simulink model "X8"  (R2020b)
settings: Solver=FixedStepAuto  StartTime=0.0  StopTime=Inf  FixedStep=1e-3  MinStep=0.0001  RelTol=1e-3  EnableMultiTasking=on
model workspace (MAT data in the model file):
  FaultMode : Simulink.Parameter (value not decoded)
values from neighbouring files (symbols this model uses):
  A = [ ... (first row only)    [calc_sys_long.m]
  C_L_delta_eInterpolation = Create_interpolation(C_L_delta_e_data,'C_L_delta_e_data')    [coeff_ctrl.m]
  F = K * (-(C_D_0 + C_D_alpha * alpha) * cos(alpha)      + (C_L_O + C_L_alpha * alpha)*sin(alpha)) - f_x    [calc_alpha.m]
  h0 = 1000    [init.m]
  input_source = 4    [runX8.m]
  input_source0 = 1    [runX8.m]
  input_step_time = 0    [runX8.m]
  J = @(v_a, omega) 2 * pi * v_a / (omega*obj.prop_diam)    [kalmanFilters.m]    (also in motor.m = 2*pi*Va/omega/prop_diam; motor_fault.m = c2 / omega)
  lat0 = 37.6205    [init.m]
  lon0 = -122.3815    [init.m]
  P = filter.P(i,i,k_0:k_1)    [filterTest.m]    (also in kalmanFilters.m = filter.P)
  p = rate(1) + wind(4)    [forces.m]    (also in forces_trim.m)
  q = rate(2) + wind(5)    [forces.m]    (also in forces_trim.m)
  r = rate(3) + wind(6)    [forces.m]    (also in forces_trim.m)
  T_elevon2ailelev = [1 1 ... (first row only)    [init.m]
  Ts = 0.01    [init.m]
  U_trim = [op.Inputs(1).u;op.Inputs(2).u;op.Inputs(3).u;op.Inputs(4).u]    [X8Trim.m]
  x0 = X_trim    [X8Trim.m]    (also in init.m = [eta_0', ny_0' zeros(1,6)]'; runX8.m = [      0                 0                    -h_ini        ; trimX8.m = [      37.5                 0                    -h_ini     )
symbols that are objects in the model workspace (value not decoded): FaultMode
undefined symbols (not defined in the file or in its folder): Friction, ia, ib, interp_C_D_alpha, interp_C_D_delta_e, interp_C_D_q, interp_C_L_alpha, interp_C_l_beta, interp_C_l_delta_a, interp_C_L_delta_e, interp_C_l_delta_r, interp_C_l_p, interp_C_L_q, interp_C_l_r, interp_C_m_alpha, interp_C_m_delta_e, interp_C_m_q, interp_C_n_beta, interp_C_n_delta_a, interp_C_n_p, interp_C_n_r, interp_C_Y_beta, interp_C_Y_delta_a, interp_C_Y_delta_r, interp_C_Y_p, interp_C_Y_r, Ion, JSBSim, Light, Lithium, Lls, MIL, Prop_param, Rascal110, Receive, Rs, Send, Standard_Devices, thetam, UDP_Protocol, wm, x0_stationary
libraries: simulink_extras x15, simulink x8, aerolibwind2 x4, sldrtlib x3, aerolibfltsims x3, aerolibactuator x3, sharedtransform x3, electricdrivelib x2, dspnetwork x1, aerolibnav x1, sharedutil x1, powerlib_meascontrol x1
(part 2 of 2)

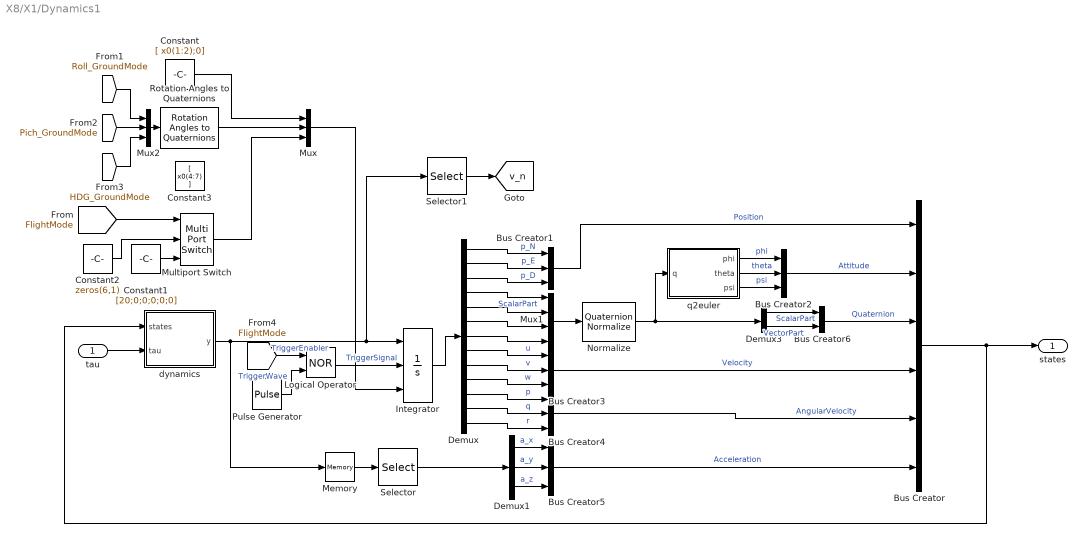
== system X8/X1/Dynamics1 ==
  tau : Inport
  Bus Creator : BusCreator  Inputs=6  OutDataTypeStr=Bus: States
  Bus Creator1 : BusCreator  Inputs=3  OutDataTypeStr=Bus: Position
  Bus Creator2 : BusCreator  Inputs=3  OutDataTypeStr=Bus: Attitude
  Bus Creator3 : BusCreator  Inputs=3  OutDataTypeStr=Bus: Velocity
  Bus Creator4 : BusCreator  Inputs=3  OutDataTypeStr=Bus: AngularVelocity
  Bus Creator5 : BusCreator  Inputs=3  OutDataTypeStr=Bus: Acceleration
  Bus Creator6 : BusCreator  Inputs=2  OutDataTypeStr=Bus: Quaternion
  Constant : Constant  Value=[ x0(1:2);0]
  Constant1 : Constant  Value=[20;0;0;0;0;0]
  Constant2 : Constant  Value=zeros(6,1)
  Constant3 : Constant  Value=[ x0(4:7) ]
  Demux : Demux  Outputs=13
  Demux1 : Demux  Outputs=3
  Demux3 : Demux  Outputs=[1,3]
  Integrator : Integrator  ExternalReset=either  InitialConditionSource=external  InitialCondition=x0_stationary(1:13)
  Logical Operator : Logic  Operator=NOR  AllPortsSameDT=off  OutDataTypeStr=boolean
  Memory : Memory
  Multiport Switch : MultiPortSwitch  DataPortOrder=Zero-based contiguous  Inputs=2  zeroidx=on
  Mux : Mux  Inputs=3
  Mux1 : Mux
  Mux2 : Mux  Inputs=3
  Normalize : sharedutil/Quaternion Normalize  aMode=aMode
      settings: SourceProductBaseCode=AE,PW,MT,UV,VE,VP
  Pulse Generator : DiscretePulseGenerator  PulseType=Time based  Period=0.2  PulseWidth=50
  Rotation Angles to Quaternions : sharedtransform/Rotation Angles to Quaternions  rotationOrder=XYZ  aMode=aMode
      settings: SourceProductBaseCode=AE,PW,MT,UV,VE,VP
  Selector : Selector  InputPortWidth=13  IndexOptions=Index vector (dialog)  Indices=8:10  OutputSizes=1
  Selector1 : Selector  InputPortWidth=13  IndexOptions=Index vector (dialog)  Indices=[1 2 3 11 12 13]  OutputSizes=1
  dynamics : MATLAB Function  TreatAsAtomicUnit=on
  q2euler : MATLAB Function  TreatAsAtomicUnit=on
  states : Outport  VectorParamsAs1DForOutWhenUnconnected=off
  tag scope: v_n=global
  wires:
  dynamics/1(y) -> Selector1/1, Integrator/1, Memory/1
  tau/1 -> dynamics/2(tau)
  Bus Creator/1 -> states/1, dynamics/1(states)
  Demux/2 -> Bus Creator1/2  "p_E"
  Demux/3 -> Bus Creator1/3  "p_D"
  Demux/1 -> Bus Creator1/1  "p_N"
  q2euler/2(theta) -> Bus Creator2/2  "theta"
  q2euler/3(psi) -> Bus Creator2/3  "psi"
  q2euler/1(phi) -> Bus Creator2/1  "phi"
  Demux/10 -> Bus Creator3/3  "w"
  Demux/8 -> Bus Creator3/1  "u"
  Demux/9 -> Bus Creator3/2  "v"
  Demux/11 -> Bus Creator4/1  "p"
  Demux/13 -> Bus Creator4/3  "r"
  Demux/12 -> Bus Creator4/2  "q"
  Bus Creator3/1 -> Bus Creator/4  "Velocity"
  Bus Creator1/1 -> Bus Creator/1  "Position"
  Bus Creator4/1 -> Bus Creator/5  "AngularVelocity"
  Bus Creator5/1 -> Bus Creator/6  "Acceleration"
  Selector/1 -> Demux1/1
  Demux1/1 -> Bus Creator5/1  "a_x"
  Demux1/2 -> Bus Creator5/2  "a_y"
  Demux1/3 -> Bus Creator5/3  "a_z"
  Demux/6 -> Mux1/3
  Demux/7 -> Mux1/4
  Demux/5 -> Mux1/2
  Normalize/1 -> q2euler/1(q), Demux3/1
  Integrator/1 -> Demux/1
  Demux3/1 -> Bus Creator6/1  "ScalarPart"
  Demux3/2 -> Bus Creator6/2  "VectorPart"
  Bus Creator6/1 -> Bus Creator/3  "Quaternion"
  Demux/4 -> Mux1/1  "ScalarPart"
  Bus Creator2/1 -> Bus Creator/2  "Attitude"
  Mux1/1 -> Normalize/1
  Memory/1 -> Selector/1
  [FlightMode] -> Multiport Switch/1
  Constant1/1 -> Multiport Switch/3
  Constant/1 -> Mux/1
  Mux2/1 -> Rotation Angles to Quaternions/1
  [Roll_GroundMode] -> Mux2/1
  [Pich_GroundMode] -> Mux2/2
  [HDG_GroundMode] -> Mux2/3
  Pulse Generator/1 -> Logical Operator/2  "TriggerWave"
  Logical Operator/1 -> Integrator/2  "TriggerSignal"
  [FlightMode] -> Logical Operator/1  "TriggerEnabler"
  Constant2/1 -> Multiport Switch/2
  Multiport Switch/1 -> Mux/3
  Mux/1 -> Integrator/3
  Rotation Angles to Quaternions/1 -> Mux/2
  Selector1/1 -> [v_n]

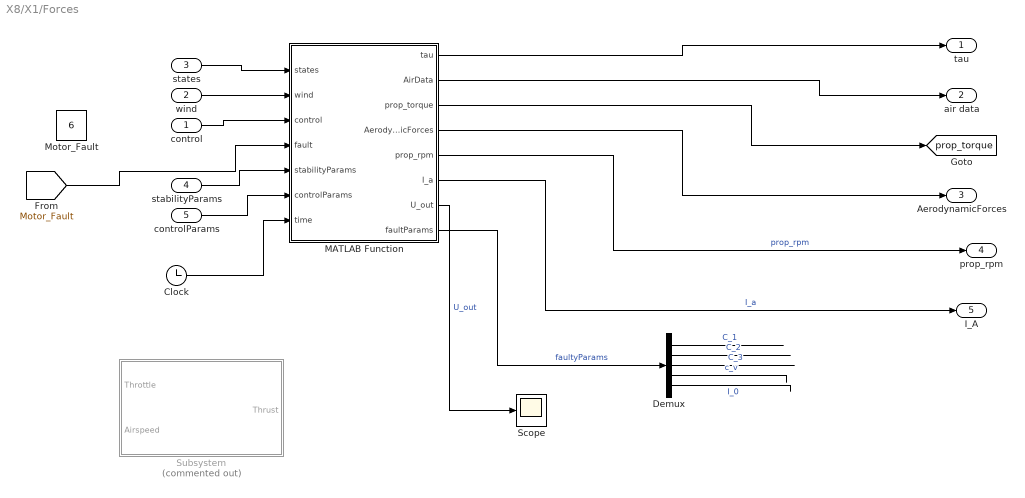
== system X8/X1/Forces ==
  control : Inport
  wind : Inport  Port=2
  states : Inport  Port=3
  stabilityParams : Inport  Port=4
  controlParams : Inport  Port=5
  Clock : Clock
  Demux : Demux  Outputs=5
  MATLAB Function : MATLAB Function  TreatAsAtomicUnit=on
  Motor_Fault : Constant  Value=6
  Scope : Scope
  Subsystem : Subsystem  Commented=on
  tau : Outport  VectorParamsAs1DForOutWhenUnconnected=off
  air data : Outport  Port=2  VectorParamsAs1DForOutWhenUnconnected=off
  AerodynamicForces : Outport  Port=3  VectorParamsAs1DForOutWhenUnconnected=off
  prop_rpm : Outport  Port=4  VectorParamsAs1DForOutWhenUnconnected=off
  I_A : Outport  Port=5  VectorParamsAs1DForOutWhenUnconnected=off
  tag scope: prop_torque=global
  wires:
  states/1 -> MATLAB Function/1(states)
  control/1 -> MATLAB Function/3(control)
  wind/1 -> MATLAB Function/2(wind)
  MATLAB Function/1(tau) -> tau/1
  MATLAB Function/3(prop_torque) -> [prop_torque]
  MATLAB Function/2(AirData) -> air data/1
  [Motor_Fault] -> MATLAB Function/4(fault)
  stabilityParams/1 -> MATLAB Function/5(stabilityParams)
  MATLAB Function/4(AerodynamicForces) -> AerodynamicForces/1
  controlParams/1 -> MATLAB Function/6(controlParams)
  MATLAB Function/5(prop_rpm) -> prop_rpm/1  "prop_rpm"
  MATLAB Function/6(I_a) -> I_A/1  "I_a"
  MATLAB Function/7(U_out) -> Scope/1  "U_out"
  Clock/1 -> MATLAB Function/7(time)
  MATLAB Function/8(faultParams) -> Demux/1  "faultyParams"
  Demux/1 -> ?  "C_1"
  Demux/2 -> ?  "C_2"
  Demux/3 -> ?  "C_3"
  Demux/4 -> ?  "c_v"
  Demux/5 -> ?  "I_0"

== system X8/X1/Terminate Function ==
  Event Listener : EventListener  DisableCoverage=on  EventType=Terminate  EventName=reset
  MATLAB Function : MATLAB Function  TreatAsAtomicUnit=on

== system X8/X1/wind model ==
  air data : Inport
  states : Inport  Port=2
  Bus Selector1 : BusSelector  OutputSignals=Va
  Bus Selector5 : BusSelector  OutputSignals=Position.p_D,Quaternion
  Dryden Wind Turbulence Model (Continuous (-q +r)) : aerolibwind2/Dryden Wind Turbulence Model  (Continuous (+q -r))  Commented=on  units=Metric (MKS)  spec=MIL-F-8785C  model=Discrete Dryden (+q -r)  W20=wind.speed  Wdeg=wind.dir  TurbProb=10^-2 - Light  L_high=533.4  Wingspan=P.b  ts=0.1  Seed=[23341 23342 23343 23344]  T_on=on
  Dryden Wind Turbulence Model (Discrete (-q +r)) : aerolibwind2/Dryden Wind Turbulence Model  (Continuous (+q -r))  units=Metric (MKS)  spec=MIL-F-8785C  model=Discrete Dryden (-q +r)  W20=3  Wdeg=wind.dir  TurbProb=10^-2 - Light  L_high=533.4  Wingspan=P.b  ts=1e-3  Seed=[23341 23342 23343 23344]  T_on=on
  Horizontal Wind Model : aerolibwind2/Horizontal Wind Model  units=Metric (MKS)  Vw_source=Internal  Vwind=3  W_source=Internal  Wdeg=wind.dir
      settings: SourceProductBaseCode=AE
  Mux : Mux  Inputs=2
  Quaternions to Direction Cosine Matrix : sharedtransform/Quaternions to  Direction Cosine Matrix  aMode=aMode
      settings: SourceProductBaseCode=AE,PW,MT,UV,VE,VP
  Sum : Sum  Inputs=|++
  Wind Shear Model : aerolibwind2/Wind Shear Model  Commented=on  units=Metric (MKS)  phase=Other  W_20=5  Wdeg=0
  down2h : Gain  Gain=-1
  gain shear wind : Gain  Commented=on  Gain=0
  gain shear wind3 : Gain
  zero wind1 : Constant  Commented=on  Value=zeros(3,1)
  wind : Outport  VectorParamsAs1DForOutWhenUnconnected=off
  wires:
  Bus Selector5/1 -> down2h/1  "<p_D>"
  Quaternions to Direction Cosine Matrix/1 -> Horizontal Wind Model/1, Dryden Wind Turbulence Model (Discrete (-q +r))/3, Wind Shear Model/2
  Bus Selector1/1 -> Dryden Wind Turbulence Model (Discrete (-q +r))/2  "<Va>"
  Bus Selector5/2 -> Quaternions to Direction Cosine Matrix/1  "<Quaternion>"
  air data/1 -> Bus Selector1/1
  states/1 -> Bus Selector5/1
  down2h/1 -> Wind Shear Model/1, Dryden Wind Turbulence Model (Discrete (-q +r))/1
  Wind Shear Model/1 -> gain shear wind/1
  Horizontal Wind Model/1 -> gain shear wind3/1
  Sum/1 -> Mux/1
  Dryden Wind Turbulence Model (Discrete (-q +r))/2 -> Mux/2
  ? -> ?
  Mux/1 -> wind/1
  gain shear wind3/1 -> Sum/1
  Dryden Wind Turbulence Model (Discrete (-q +r))/1 -> Sum/2

== system X8/X1/Actuators2/Actuator dynamics ==
  Demanded R elevon deflection : Inport
  "Demanded L elevon deflection " : Inport  Port=2
  Demanded rudder deflection1 : Inport  Port=3
  Demanded motor speed : Inport  Port=4
  Prop torque : Inport  Port=5
  Motor : Subsystem  Commented=through  mask{T=0.2, X0=x0(18)}
      mask prompts: T "Time constant"; X0 "Initial condition"
      mask DialogControl DescGroupVar Prompt: Motor model
      mask DialogControl DescTextVar Prompt: Simple first order motor model
  Saturation : Saturate  UpperLimit=P.aileronMax  LowerLimit=P.aileronMin
  Saturation1 : Saturate  UpperLimit=P.aileronMax  LowerLimit=P.aileronMin
  Servo and control surface dynamics L : aerolibactuator/Nonlinear Second-Order Actuator  Commented=through  wn_fin=P.servo.omega0  z_fin=P.servo.zeta  fin_max=P.servo.max_rad  fin_min=P.servo.min_rad  fin_maxrate=P.servo.rate_lim  fin_act_0=x0(16)  fin_act_vel=x0(17)
      settings: SourceProductBaseCode=AE
  Servo and control surface dynamics R : aerolibactuator/Nonlinear Second-Order Actuator  Commented=through  wn_fin=P.servo.omega0  z_fin=P.servo.zeta  fin_max=P.servo.max_rad  fin_min=P.servo.min_rad  fin_maxrate=P.servo.rate_lim  fin_act_0=x0(14)  fin_act_vel=x0(15)
      settings: SourceProductBaseCode=AE
  Servo and control surface dynamics1 : aerolibactuator/Nonlinear Second-Order Actuator  Commented=through  wn_fin=P.servo.omega0  z_fin=P.servo.zeta  fin_max=P.servo.max_rad  fin_min=P.servo.min_rad  fin_maxrate=P.servo.rate_lim  fin_act_0=P.servo.pos0  fin_act_vel=P.servo.rate0
      settings: SourceProductBaseCode=AE
  Subsystem : Subsystem  Commented=on
  Applied R elevon : Outport  VectorParamsAs1DForOutWhenUnconnected=off
  Applied L elevon : Outport  Port=2  VectorParamsAs1DForOutWhenUnconnected=off
  Applied rudder : Outport  Port=3  VectorParamsAs1DForOutWhenUnconnected=off
  Applied motor speed : Outport  Port=4  VectorParamsAs1DForOutWhenUnconnected=off
  wires:
  Servo and control surface dynamics R/1 -> Saturation/1
  Motor/1(n) -> Applied motor speed/1
  Servo and control surface dynamics1/1 -> Applied rudder/1
  Servo and control surface dynamics L/1 -> Saturation1/1
  Demanded rudder deflection1/1 -> Servo and control surface dynamics1/1
  Demanded motor speed/1 -> Motor/1(n_d)
  Demanded R elevon deflection/1 -> Servo and control surface dynamics R/1
  "Demanded L elevon deflection "/1 -> Servo and control surface dynamics L/1
  Saturation/1 -> Applied R elevon/1
  Saturation1/1 -> Applied L elevon/1

== system X8/X1/Actuators2/PWM lookup ==
  Rservo PWM : Inport
  Lservo : Inport  Port=2
  Rudder : Inport  Port=3
  thr pwm : Inport  Port=4
  1-D Lookup Table1 : Lookup_n-D  Commented=through  NumberOfTableDimensions=1  BreakpointsForDimension1=|  Table=|  InternalRulePriority=Speed  RndMeth=Simplest  InputSameDT=on
      BreakpointsForDimension1=|
      | [-20
      | -15
      | -10
      | 15
      | 20
      | 21.6]
      Table=|
      | [1260
      | 1400
      | 1480
      | 1770
      | 1880
      | 1920]
  1-D Lookup Table2 : Lookup_n-D  Commented=through  NumberOfTableDimensions=1  BreakpointsForDimension1=|  Table=|  InternalRulePriority=Speed  RndMeth=Simplest  InputSameDT=on
      BreakpointsForDimension1=|
      | [-20
      | -15
      | -10
      | 15
      | 20
      | 21.6]
      Table=|
      | [1260
      | 1400
      | 1480
      | 1770
      | 1880
      | 1920]
  1-D Lookup Table3 : Lookup_n-D  Commented=through  NumberOfTableDimensions=1  BreakpointsForDimension1=|  Table=|  InternalRulePriority=Speed  RndMeth=Simplest  InputSameDT=on
      BreakpointsForDimension1=|
      | [-20
      | -15
      | -10
      | 15
      | 20
      | 21.6]
      Table=|
      | [1260
      | 1400
      | 1480
      | 1770
      | 1880
      | 1920]
  Saturation{,1..3} (4 alike) : Saturate  Commented=through  UpperLimit=P.pwmMax  LowerLimit=P.pwmMin
  pwm to thrust : Lookup_n-D  Commented=through  NumberOfTableDimensions=1  BreakpointsForDimension1=[1000 2000]  Table=[0 1]  InternalRulePriority=Speed  RndMeth=Simplest  InputSameDT=on
  Rservo deflection : Outport  VectorParamsAs1DForOutWhenUnconnected=off
  Lservo deflection : Outport  Port=2  VectorParamsAs1DForOutWhenUnconnected=off
  rud deflection : Outport  Port=3  VectorParamsAs1DForOutWhenUnconnected=off
  thrust : Outport  Port=4  VectorParamsAs1DForOutWhenUnconnected=off
  wires:
  Saturation2/1 -> 1-D Lookup Table2/1
  1-D Lookup Table1/1 -> Rservo deflection/1
  pwm to thrust/1 -> thrust/1
  Rservo PWM/1 -> Saturation/1
  thr pwm/1 -> Saturation3/1
  Saturation1/1 -> 1-D Lookup Table3/1
  Saturation3/1 -> pwm to thrust/1
  Saturation/1 -> 1-D Lookup Table1/1
  Lservo/1 -> Saturation1/1
  Rudder/1 -> Saturation2/1
  1-D Lookup Table2/1 -> rud deflection/1
  1-D Lookup Table3/1 -> Lservo deflection/1

== system X8/X1/Actuators2/Scale to [-1..1] ==
  deflection : Inport
  Gain : Gain  Gain=1/P.aileronMax
  Saturation : Saturate  UpperLimit=1  LowerLimit=-1
  scaled deflection : Outport  VectorParamsAs1DForOutWhenUnconnected=off
  wires:
  deflection/1 -> Gain/1
  Gain/1 -> Saturation/1
  Saturation/1 -> scaled deflection/1

== system X8/X1/Actuators2/Scale to [0..1] ==
  prop speed : Inport
  Gain : Gain  Commented=through  Gain=1/P.motor.omega_max
  Saturation : Saturate  UpperLimit=1  LowerLimit=0
  scaled prop speed : Outport  VectorParamsAs1DForOutWhenUnconnected=off
  wires:
  prop speed/1 -> Gain/1
  Gain/1 -> Saturation/1
  Saturation/1 -> scaled prop speed/1

== system X8/X1/Calculate Stability Parameters/Subsystem ==
  alpha : Inport
  icing : Inport  Port=2
  2-D Lookup Table : Lookup_n-D  DataSpecification=Lookup table object  LookupTableObject=C_L_aInterpolation  BreakpointsForDimension1=C_L_delta_eInterpolation.Points(:,1)  BreakpointsForDimension2=C_L_delta_eInterpolation.Points(:,2)  BreakpointsForDimension1FirstPoint=4  BreakpointsForDimension2FirstPoint=2  IndexSearchMethod=Linear search  Table=C_L_delta_eInterpolation.Values  ExtrapMethod=Clip  InternalRulePriority=Speed  RndMeth=Simplest  InputSameDT=on
      settings: InputPortMap=u0,u1
  2-D Lookup Table1 : Lookup_n-D  DataSpecification=Lookup table object  LookupTableObject=C_L_qInterpolation  BreakpointsForDimension1=C_L_delta_eInterpolation.Points(:,1)  BreakpointsForDimension2=C_L_delta_eInterpolation.Points(:,2)  BreakpointsForDimension1FirstPoint=4  BreakpointsForDimension2FirstPoint=2  IndexSearchMethod=Linear search  Table=C_L_delta_eInterpolation.Values  InternalRulePriority=Speed  RndMeth=Simplest  InputSameDT=on
      settings: InputPortMap=u0,u1
  2-D Lookup Table2 : Lookup_n-D  DataSpecification=Lookup table object  LookupTableObject=C_D_aInterpolation  BreakpointsForDimension1=C_L_delta_eInterpolation.Points(:,1)  BreakpointsForDimension2=C_L_delta_eInterpolation.Points(:,2)  BreakpointsForDimension1FirstPoint=4  BreakpointsForDimension2FirstPoint=2  IndexSearchMethod=Linear search  Table=C_L_delta_eInterpolation.Values  InternalRulePriority=Speed  RndMeth=Simplest  InputSameDT=on
      settings: InputPortMap=u0,u1
  2-D Lookup Table3 : Lookup_n-D  DataSpecification=Lookup table object  LookupTableObject=C_D_qInterpolation  BreakpointsForDimension1=C_L_delta_eInterpolation.Points(:,1)  BreakpointsForDimension2=C_L_delta_eInterpolation.Points(:,2)  BreakpointsForDimension1FirstPoint=4  BreakpointsForDimension2FirstPoint=2  IndexSearchMethod=Linear search  Table=C_L_delta_eInterpolation.Values  InternalRulePriority=Speed  RndMeth=Simplest  InputSameDT=on
      settings: InputPortMap=u0,u1
  2-D Lookup Table4 : Lookup_n-D  DataSpecification=Lookup table object  LookupTableObject=C_m_qInterpolation  BreakpointsForDimension1=C_L_delta_eInterpolation.Points(:,1)  BreakpointsForDimension2=C_L_delta_eInterpolation.Points(:,2)  BreakpointsForDimension1FirstPoint=4  BreakpointsForDimension2FirstPoint=2  IndexSearchMethod=Linear search  Table=C_L_delta_eInterpolation.Values  InternalRulePriority=Speed  RndMeth=Simplest  InputSameDT=on
      settings: InputPortMap=u0,u1
  2-D Lookup Table5 : Lookup_n-D  DataSpecification=Lookup table object  LookupTableObject=C_m_aInterpolation  BreakpointsForDimension1=C_L_delta_eInterpolation.Points(:,1)  BreakpointsForDimension2=C_L_delta_eInterpolation.Points(:,2)  BreakpointsForDimension1FirstPoint=4  BreakpointsForDimension2FirstPoint=2  IndexSearchMethod=Linear search  Table=C_L_delta_eInterpolation.Values  InternalRulePriority=Speed  RndMeth=Simplest  InputSameDT=on
      settings: InputPortMap=u0,u1
  Bus Creator : BusCreator  Inputs=6
  Out1 : Outport  VectorParamsAs1DForOutWhenUnconnected=off
  wires:
  Bus Creator/1 -> Out1/1
  2-D Lookup Table/1 -> Bus Creator/1  "C_L_alpha"
  alpha/1 -> 2-D Lookup Table4/1, 2-D Lookup Table5/1, 2-D Lookup Table3/1, 2-D Lookup Table2/1, 2-D Lookup Table1/1, 2-D Lookup Table/1
  icing/1 -> 2-D Lookup Table3/2, 2-D Lookup Table5/2, 2-D Lookup Table4/2, 2-D Lookup Table2/2, 2-D Lookup Table1/2, 2-D Lookup Table/2
  2-D Lookup Table1/1 -> Bus Creator/2  "C_L_q"
  2-D Lookup Table2/1 -> Bus Creator/3  "C_D_alpha"
  2-D Lookup Table3/1 -> Bus Creator/4  "C_D_q"
  2-D Lookup Table5/1 -> Bus Creator/5  "C_m_alpha"
  2-D Lookup Table4/1 -> Bus Creator/6  "C_m_q"

== system X8/X1/Calculate Stability Parameters/Subsystem1 ==
  beta : Inport
  icing : Inport  Port=2
  2-D Lookup Table : Lookup_n-D  DataSpecification=Lookup table object  LookupTableObject=C_Y_bInterpolation  BreakpointsForDimension1=C_L_delta_eInterpolation.Points(:,1)  BreakpointsForDimension2=C_L_delta_eInterpolation.Points(:,2)  BreakpointsForDimension1FirstPoint=4  BreakpointsForDimension2FirstPoint=2  IndexSearchMethod=Linear search  Table=C_L_delta_eInterpolation.Values  InternalRulePriority=Speed  RndMeth=Simplest  InputSameDT=on
      settings: InputPortMap=u0,u1
  2-D Lookup Table1 : Lookup_n-D  DataSpecification=Lookup table object  LookupTableObject=C_Y_pInterpolation  BreakpointsForDimension1=C_L_delta_eInterpolation.Points(:,1)  BreakpointsForDimension2=C_L_delta_eInterpolation.Points(:,2)  BreakpointsForDimension1FirstPoint=4  BreakpointsForDimension2FirstPoint=2  IndexSearchMethod=Linear search  Table=C_L_delta_eInterpolation.Values  InternalRulePriority=Speed  RndMeth=Simplest  InputSameDT=on
      settings: InputPortMap=u0,u1
  2-D Lookup Table2 : Lookup_n-D  DataSpecification=Lookup table object  LookupTableObject=C_Y_rInterpolation  BreakpointsForDimension1=C_L_delta_eInterpolation.Points(:,1)  BreakpointsForDimension2=C_L_delta_eInterpolation.Points(:,2)  BreakpointsForDimension1FirstPoint=4  BreakpointsForDimension2FirstPoint=2  IndexSearchMethod=Linear search  Table=C_L_delta_eInterpolation.Values  InternalRulePriority=Speed  RndMeth=Simplest  InputSameDT=on
      settings: InputPortMap=u0,u1
  2-D Lookup Table3 : Lookup_n-D  DataSpecification=Lookup table object  LookupTableObject=C_l_bInterpolation  BreakpointsForDimension1=C_L_delta_eInterpolation.Points(:,1)  BreakpointsForDimension2=C_L_delta_eInterpolation.Points(:,2)  BreakpointsForDimension1FirstPoint=4  BreakpointsForDimension2FirstPoint=2  IndexSearchMethod=Linear search  Table=C_L_delta_eInterpolation.Values  InternalRulePriority=Speed  RndMeth=Simplest  InputSameDT=on
      settings: InputPortMap=u0,u1
  2-D Lookup Table4 : Lookup_n-D  DataSpecification=Lookup table object  LookupTableObject=C_l_rInterpolation  BreakpointsForDimension1=C_L_delta_eInterpolation.Points(:,1)  BreakpointsForDimension2=C_L_delta_eInterpolation.Points(:,2)  BreakpointsForDimension1FirstPoint=4  BreakpointsForDimension2FirstPoint=2  IndexSearchMethod=Linear search  Table=C_L_delta_eInterpolation.Values  InternalRulePriority=Speed  RndMeth=Simplest  InputSameDT=on
      settings: InputPortMap=u0,u1
  2-D Lookup Table5 : Lookup_n-D  DataSpecification=Lookup table object  LookupTableObject=C_l_pInterpolation  BreakpointsForDimension1=C_L_delta_eInterpolation.Points(:,1)  BreakpointsForDimension2=C_L_delta_eInterpolation.Points(:,2)  BreakpointsForDimension1FirstPoint=4  BreakpointsForDimension2FirstPoint=2  IndexSearchMethod=Linear search  Table=C_L_delta_eInterpolation.Values  InternalRulePriority=Speed  RndMeth=Simplest  InputSameDT=on
      settings: InputPortMap=u0,u1
  2-D Lookup Table6 : Lookup_n-D  DataSpecification=Lookup table object  LookupTableObject=C_n_bInterpolation  BreakpointsForDimension1=C_L_delta_eInterpolation.Points(:,1)  BreakpointsForDimension2=C_L_delta_eInterpolation.Points(:,2)  BreakpointsForDimension1FirstPoint=4  BreakpointsForDimension2FirstPoint=2  IndexSearchMethod=Linear search  Table=C_L_delta_eInterpolation.Values  InternalRulePriority=Speed  RndMeth=Simplest  InputSameDT=on
      settings: InputPortMap=u0,u1
  2-D Lookup Table7 : Lookup_n-D  DataSpecification=Lookup table object  LookupTableObject=C_n_pInterpolation  BreakpointsForDimension1=C_L_delta_eInterpolation.Points(:,1)  BreakpointsForDimension2=C_L_delta_eInterpolation.Points(:,2)  BreakpointsForDimension1FirstPoint=4  BreakpointsForDimension2FirstPoint=2  IndexSearchMethod=Linear search  Table=C_L_delta_eInterpolation.Values  InternalRulePriority=Speed  RndMeth=Simplest  InputSameDT=on
      settings: InputPortMap=u0,u1
  2-D Lookup Table8 : Lookup_n-D  DataSpecification=Lookup table object  LookupTableObject=C_n_rInterpolation  BreakpointsForDimension1=C_L_delta_eInterpolation.Points(:,1)  BreakpointsForDimension2=C_L_delta_eInterpolation.Points(:,2)  BreakpointsForDimension1FirstPoint=4  BreakpointsForDimension2FirstPoint=2  IndexSearchMethod=Linear search  Table=C_L_delta_eInterpolation.Values  InternalRulePriority=Speed  RndMeth=Simplest  InputSameDT=on
      settings: InputPortMap=u0,u1
  Bus Creator : BusCreator  Inputs=9
  Out1 : Outport  VectorParamsAs1DForOutWhenUnconnected=off
  wires:
  Bus Creator/1 -> Out1/1
  icing/1 -> 2-D Lookup Table/2, 2-D Lookup Table6/2, 2-D Lookup Table7/2, 2-D Lookup Table8/2, 2-D Lookup Table4/2, 2-D Lookup Table5/2, 2-D Lookup Table3/2, 2-D Lookup Table2/2, 2-D Lookup Table1/2
  2-D Lookup Table1/1 -> Bus Creator/2  "C_Y_p"
  beta/1 -> 2-D Lookup Table5/1, 2-D Lookup Table8/1, 2-D Lookup Table7/1, 2-D Lookup Table6/1, 2-D Lookup Table4/1, 2-D Lookup Table3/1, 2-D Lookup Table2/1, 2-D Lookup Table1/1, 2-D Lookup Table/1
  2-D Lookup Table2/1 -> Bus Creator/3  "C_Y_r"
  2-D Lookup Table/1 -> Bus Creator/1  "C_Y_beta"
  2-D Lookup Table5/1 -> Bus Creator/5  "C_l_p"
  2-D Lookup Table3/1 -> Bus Creator/4  "C_l_beta"
  2-D Lookup Table4/1 -> Bus Creator/6  "C_l_r"
  2-D Lookup Table6/1 -> Bus Creator/7  "C_n_beta"
  2-D Lookup Table7/1 -> Bus Creator/8  "C_n_p"
  2-D Lookup Table8/1 -> Bus Creator/9  "C_n_r"

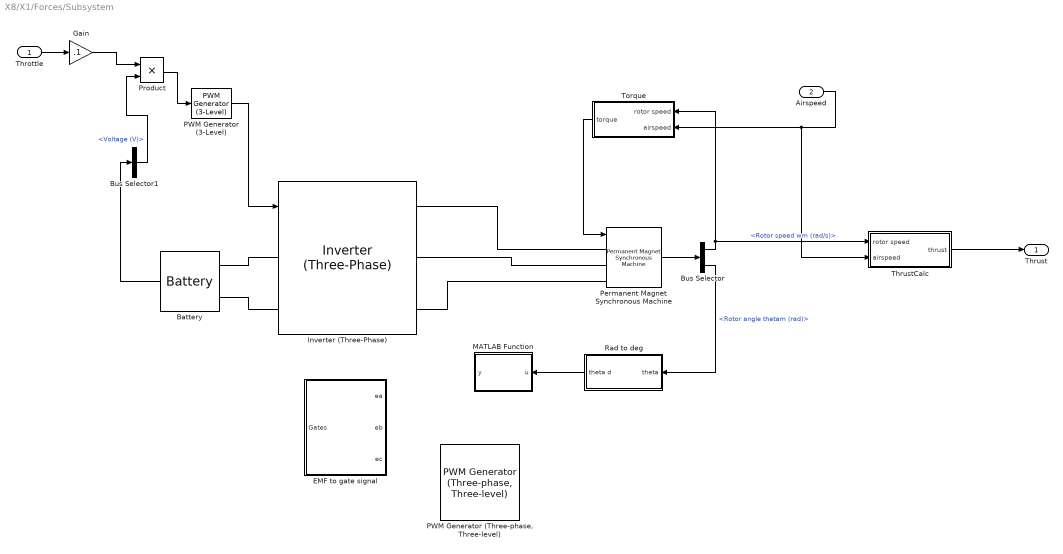
== system X8/X1/Forces/Subsystem ==
  Throttle : Inport
  Airspeed : Inport  Port=2
  Battery : electricdrivelib/Extra Sources/Battery  BatType=Lithium-Ion  ShowTempParam=off  ThermalPreset=no  ShowAgeParam=off  NomV=14  NomQ=1000  SOC=100  Batt_Tr=30  PresetModel=on  MaxQ=1000  MinV=10.5  FullV=16.2958  Dis_rate=434.7826  R=0.00014  Normal_OP=904.3478  expZone="[15.1254      49.1304]"  current=[6.5 13 32.5]  Units=Time  Tci=20  NomT=20  T2=-30  MaxQ2=4.8  FullV2=7.1  Normal_OP2=5.655  expZone2="[6.58           1]"  Rca=0.6  ti=2000  Dp=0  Neq0=0  Tsim=1e6  Ta1=25  Qeol=5.4*0.9  Reol=0.013333*1.2  Char_age=[2.3478, 3]  Dis_age=[2.3478, 10]  N1=1500  N2=10500  N3=1000  N4=1400  Ta2=45  N5=950
  Bus Selector : BusSelector  OutputSignals=Rotor speed wm (rad/s),Rotor angle thetam (rad)
  Bus Selector1 : BusSelector  OutputSignals=Voltage (V)
  EMF to gate signal : Subsystem
  Gain : Gain  Gain=.1
  Inverter (Three-Phase) : electricdrivelib/Fundamental Drive Blocks/Inverter (Three-Phase)  LabelModeActiveChoice=Detailed  detailLevel=Detailed  driveType=Brushless DC  Ts=2e-6  SnubberResistance=10e3  SnubberCapacitance=inf  Device=MOSFET / Diodes  Ron=1e-3  ForwardVoltages=[1.2,1.2]  GTOparameters=[1e-6,2e-6]  IGBTparameters=[1e-6,2e-6]  Measurements=All voltages and currents  converterType=Inverter  SourceFrequency=60  ReferenceFrame=Rotor  dqInductances=[8.5e-3,8.5e-3]  Inductance=8.5e-3  Ls=0  Resistance=0.2  Flux=0.175  Stator_sm=[2.01e-3,4.289e-4,4.477e-3,1.354e-3]  Stator_im=[14.85e-3,0.3027e-3]  Rotor=[9.295e-3,0.3027e-3]  Lm=10.46e-3  p=4
      settings: AttributesFormatString=%<BlockChoice>  SourceProductBaseCode=PS
  MATLAB Function : MATLAB Function  TreatAsAtomicUnit=on
  PWM Generator (3-Level) : powerlib_meascontrol/Pulse & Signal Generators/PWM Generator (3-Level)  ModulatorType=Three-phase bridge (12 pulses)  ModulatorMode=Unsynchronized  nF=27  Fc=27*60  ModulatingSignals=off  m=0.8  Freq=60  Phase=0  Ts=0
      settings: SourceProductBaseCode=PS
  "PWM Generator (Three-phase, Three-level)" : pePwmGeneratorThreeLevel/PWM Generator (Three-phase, Three-level)  CPWMMode=SPWM: sinusoidal PWM  fsw=1e3  Ts=5e-5
      settings: SourceProductBaseCode=PS  SamplingMode=Natural
  Permanent Magnet Synchronous Machine : powerlib/Machines/Permanent Magnet Synchronous Machine  NbPhases=3  FluxDistribution=Trapezoidal  RotorType=Round  MechanicalLoad=Torque Tm  PresetModel=No  ShowDetailedParameters=on  MeasurementBus=off  Resistance=Rs  Inductance=Lls  dqInductances=[8.5e-3,8.5e-3]  La=0.000835  MachineConstant=Flux linkage established by magnets (V.s)  Flux=0.175  VoltageCst=146.6077  TorqueCst=1.4  Flat=Flat  Mechanical=[J,Friction,p]  PolePairs=4  InitialConditions=[wm,thetam,ia,ib]  InitialConditions5ph=[0 0 0 0 0 0]  RefAngle=90 degrees behind phase A axis (modified Park)  IterativeDiscreteModel=Trapezoidal non iterative  TsBlock=-1  TsPowergui=0
  Product : Product
  Rad to deg : Subsystem
  ThrustCalc : Subsystem
  Torque : Subsystem
  Thrust : Outport  VectorParamsAs1DForOutWhenUnconnected=off
  wires:
  Permanent Magnet Synchronous Machine/1 -> Bus Selector/1
  Bus Selector/1 -> Torque/1(rotor speed), ThrustCalc/1(rotor speed)  "<Rotor speed wm (rad/s)>"
  PWM Generator (3-Level)/1 -> Inverter (Three-Phase)/1
  Battery/1 -> Bus Selector1/1
  Product/1 -> PWM Generator (3-Level)/1
  Bus Selector1/1 -> Product/2  "<Voltage (V)>"
  Throttle/1 -> Gain/1
  Gain/1 -> Product/1
  Torque/1(torque) -> Permanent Magnet Synchronous Machine/1
  ThrustCalc/1(thrust) -> Thrust/1
  Airspeed/1 -> ThrustCalc/2(airspeed), Torque/2(airspeed)
  Bus Selector/2 -> Rad to deg/1(theta)  "<Rotor angle thetam (rad)>"
  Rad to deg/1(theta d) -> MATLAB Function/1(u)
  connections:
  Battery/LConn1 -- Inverter (Three-Phase)/LConn1
  Battery/LConn2 -- Inverter (Three-Phase)/LConn2
  Inverter (Three-Phase)/RConn1 -- Permanent Magnet Synchronous Machine/LConn1
  Inverter (Three-Phase)/RConn2 -- Permanent Magnet Synchronous Machine/LConn2
  Inverter (Three-Phase)/RConn3 -- Permanent Magnet Synchronous Machine/LConn3

== system X8/X1/Actuators2/Actuator dynamics/Motor ==
  n_d : Inport
  1/T : Gain  Gain=1/T
  Integrator : Integrator  InitialCondition=X0  ContinuousStateAttributes='throttle'
  Sum : Sum  Inputs=|+-
  n : Outport  VectorParamsAs1DForOutWhenUnconnected=off
  wires:
  Integrator/1 -> n/1, Sum/2
  n_d/1 -> Sum/1
  Sum/1 -> 1/T/1
  1/T/1 -> Integrator/1

== system X8/X1/Actuators2/Actuator dynamics/Subsystem ==
  In1 : Inport
  In2 : Inport  Port=2
  1/J_prop : Gain  Gain=1/P.J_prop  SaturateOnIntegerOverflow=on  OutDataTypeStr=Inherit: Same as input  ParamDataTypeStr=Inherit: Same as input
  Demand limits : Saturate  UpperLimit=1  LowerLimit=0
  Integrator : Integrator  InitialCondition=0.5
  Kp : Gain  SaturateOnIntegerOverflow=on  OutDataTypeStr=Inherit: Same as input  ParamDataTypeStr=Inherit: Same as input
  Kp1 : Gain  Gain=-1  SaturateOnIntegerOverflow=on  OutDataTypeStr=Inherit: Same as input  ParamDataTypeStr=Inherit: Same as input
  Sum2 : Sum  Inputs=-+|  InputSameDT=on  SaturateOnIntegerOverflow=on  OutDataTypeStr=Inherit: Same as first input
  Sum3 : Sum  Inputs=|+-  InputSameDT=on  SaturateOnIntegerOverflow=on  OutDataTypeStr=Inherit: Same as first input
  Torque limit : Saturate  UpperLimit=P.motor.torque_max  LowerLimit=0  ZeroCross=off
  Transport Delay : TransportDelay  DelayTime=0.001  PadeOrder=1
  Applied motor speed : Outport  VectorParamsAs1DForOutWhenUnconnected=off
  wires:
  Demand limits/1 -> Sum3/1
  Sum3/1 -> Kp/1
  Integrator/1 -> Applied motor speed/1, Sum3/2
  Torque limit/1 -> Sum2/2
  Sum2/1 -> 1/J_prop/1
  1/J_prop/1 -> Integrator/1
  Kp/1 -> Torque limit/1
  In1/1 -> Kp1/1
  In2/1 -> Transport Delay/1
  Transport Delay/1 -> Demand limits/1
  Kp1/1 -> Sum2/1

== system X8/X1/Forces/Subsystem/EMF to gate signal ==
  ea : Inport
  eb : Inport  Port=2
  ec : Inport  Port=3
  Compare To Zero : simulink/Logic and Bit Operations/Compare To Zero  relop=>  OutDataTypeStr=boolean  ZeroCross=off
  Compare To Zero1 : simulink/Logic and Bit Operations/Compare To Zero  relop=<  OutDataTypeStr=boolean  ZeroCross=off
  Compare To Zero2 : simulink/Logic and Bit Operations/Compare To Zero  relop=>  OutDataTypeStr=boolean  ZeroCross=off
  Compare To Zero3 : simulink/Logic and Bit Operations/Compare To Zero  relop=<  OutDataTypeStr=boolean  ZeroCross=off
  Compare To Zero4 : simulink/Logic and Bit Operations/Compare To Zero  relop=>  OutDataTypeStr=boolean  ZeroCross=off
  Compare To Zero5 : simulink/Logic and Bit Operations/Compare To Zero  relop=<  OutDataTypeStr=boolean  ZeroCross=off
  Mux3 : Mux  Inputs=6
  Gates : Outport  VectorParamsAs1DForOutWhenUnconnected=off
  wires:
  Mux3/1 -> Gates/1
  ea/1 -> Compare To Zero/1, Compare To Zero1/1
  eb/1 -> Compare To Zero2/1, Compare To Zero3/1
  ec/1 -> Compare To Zero4/1, Compare To Zero5/1
  Compare To Zero/1 -> Mux3/1
  Compare To Zero1/1 -> Mux3/2
  Compare To Zero2/1 -> Mux3/3
  Compare To Zero3/1 -> Mux3/4
  Compare To Zero4/1 -> Mux3/5
  Compare To Zero5/1 -> Mux3/6

== system X8/X1/Forces/Subsystem/Rad to deg ==
  theta : Inport
  Trigonometric Function : Trigonometry
  Trigonometric Function1 : Trigonometry  Operator=cos
  Trigonometric Function2 : Trigonometry  Operator=atan2
  rad2deg : Gain  Gain=180/pi  SaturateOnIntegerOverflow=on  OutDataTypeStr=Inherit: Same as input  ParamDataTypeStr=Inherit: Same as input
  theta d : Outport  VectorParamsAs1DForOutWhenUnconnected=off
  wires:
  theta/1 -> Trigonometric Function/1, Trigonometric Function1/1
  Trigonometric Function/1 -> Trigonometric Function2/1
  Trigonometric Function1/1 -> Trigonometric Function2/2
  Trigonometric Function2/1 -> rad2deg/1
  rad2deg/1 -> theta d/1

== system X8/X1/Forces/Subsystem/ThrustCalc ==
  rotor speed : Inport
  airspeed : Inport  Port=2
  Divide : Product  Inputs=*/
  Divide1 : Product  Inputs=**
  Gain : Gain  Gain=2*pi
  Gain1 : Gain  Gain=Prop_param.C_T_0
  Gain2 : Gain  Gain=Prop_param.C_T_J
  Math Function : Math  Operator=square  SignedPower=on  SaturateOnIntegerOverflow=on
  Sum : Sum
  thrust : Outport  VectorParamsAs1DForOutWhenUnconnected=off
  wires:
  rotor speed/1 -> Math Function/1, Divide/2
  airspeed/1 -> Gain/1
  Gain/1 -> Divide/1
  Divide/1 -> Divide1/1  "J"
  Sum/1 -> thrust/1
  Math Function/1 -> Divide1/2, Gain1/1
  Divide1/1 -> Gain2/1  "J"
  Gain2/1 -> Sum/1
  Gain1/1 -> Sum/2

== system X8/X1/Forces/Subsystem/Torque ==
  rotor speed : Inport
  airspeed : Inport  Port=2
  Derivative : Derivative
  Divide : Product  Inputs=*/
  Divide1 : Product  Inputs=**
  Gain : Gain  Gain=2*pi
  Gain1 : Gain  Gain=Prop_param.C_W_0
  Gain2 : Gain  Gain=Prop_param.C_W_J
  Gain3 : Gain  Gain=Prop_param.c_v
  Gain4 : Gain  Gain=Prop_param.J
  Math Function : Math  Operator=square  SignedPower=on  SaturateOnIntegerOverflow=on
  Sum : Sum  Inputs=++++
  torque : Outport  VectorParamsAs1DForOutWhenUnconnected=off
  wires:
  rotor speed/1 -> Derivative/1, Math Function/1, Gain3/1, Divide/2
  airspeed/1 -> Gain/1
  Gain/1 -> Divide/1
  Divide/1 -> Divide1/1  "J"
  Sum/1 -> torque/1
  Math Function/1 -> Divide1/2, Gain1/1
  Gain1/1 -> Sum/3
  Divide1/1 -> Gain2/1  "J"
  Gain2/1 -> Sum/2
  Gain3/1 -> Sum/1
  Derivative/1 -> Gain4/1
  Gain4/1 -> Sum/4

== matlab function X8/MATLAB Function ==
  data: t input; icing output
function icing = fcn(t)
    % Some icing model. 
    % icing = 0..1 
    
    NOICE_PERIOD = 30;
    ICING_TIME = 30;
    MAX_ICING = 1; 
    
    if t < NOICE_PERIOD
        icing = 0; 
    elseif t < NOICE_PERIOD + ICING_TIME
        icing = MAX_ICING * (t - NOICE_PERIOD) / ICING_TIME; 
    else
        icing = MAX_ICING; 
    end
end

== matlab function X8/X1/Forces/Subsystem/MATLAB Function ==
  data: u input; y output
function y=emfg(u)
if (u>-180)&&(u<=-120)
    y=[-1;0;1];
elseif(u>-120)&&(u<=-60)
    y=[0;-1;1];
elseif(u>-60)&&(u<=0)
    y=[1;-1;0];
elseif(u>0)&&(u<=60)
    y=[1;0;-1];
elseif(u>60)&&(u<=120)
    y=[0;1;-1];
elseif(u>120)&&(u<=180)
    y=[-1;1;0];
end
y =[y(1)>0;y(1)<0;y(2)>0;y(2)<0;y(3)>0;y(3)<0];

== matlab function X8/X1/Send Dune Airflow1 ==
  settings: updateMethod=DISCRETE  sampleTime=0.1
  data: Va input; AoA input; SSA input; wind_n input
function rcv_airflow(Va,AoA,SSA,wind_n)
coder.extrinsic('-sync:on','send_airflow_dune');
send_airflow_dune(Va,AoA,SSA,wind_n,0);

== matlab function X8/Motor Fault ==
  settings: updateMethod=DISCRETE
  data: model input; y output; mode input
function y  = fcn(model, mode)
    y = mode * model;
end

== matlab function X8/X1/Terminate Function/MATLAB Function ==
function fcn()
coder.extrinsic('-sync:on','rcv_airflow_dune');
coder.extrinsic('-sync:on','send_airflow_dune');
send_airflow_dune(0,0,0,1);
[~,~,~]=rcv_airflow_dune(1);

end

== matlab function X8/Ardupilot SITL receive/MATLAB Function ==
  data: motors output
function motors = fcn()
motors = zeros(16 ,1);
coder.extrinsic('-sync:on','simReceive');
motors = simReceive();
end

== matlab function X8/Ardupilot SITL send/MATLAB Function ==
  data: Va input; u_r output; alpha input; beta input
function u_r = fcn(Va,alpha,beta)

u_r = Va*cos(alpha)*cos(beta);

== matlab function X8/Ardupilot SITL send/MATLAB Function1 ==
  data: u input; y output
function y  = fcn(u)

y = Rquat(u);

== matlab function X8/Ardupilot SITL send/q2Rxyc ==
  data: q input; Rxy output
function Rxy  = fcn(q)
%#codegen
[phi,theta,~] = q2euler(q);

sp = sin(phi);
cp = cos(phi);
ct = cos(theta);
tt = tan(theta);

Rxy=[1 sp*tt cp*tt;...
     0 cp -sp; ...
     0 sp/ct cp/ct];
end

== matlab function X8/Mission Planner/Altitude Command ==
  settings: updateMethod=DISCRETE
  data: time input; y output
function y = fcn(time)
%#codegen
% persistent temp
% % if isempty(temp)
% %     temp=100;
% % end

% Fly a steop function and a sawtooth with low climb rate

CLIMB_RATE = 1; % m/s
STEP_SIZE = 50; % m 
ALT_MIN = 100; 
TIME_STEP = 50; %s
PERIOD = 5 * TIME_STEP;

if mod(time, PERIOD) < TIME_STEP
    y = ALT_MIN;
elseif mod(time, PERIOD) < 2 * TIME_STEP
    y = ALT_MIN + STEP_SIZE;
elseif mod(time, PERIOD) < 3 * TIME_STEP
    y = ALT_MIN; 
elseif mod(time, PERIOD) < 4 * TIME_STEP
    y = (mod(time, PERIOD) - 3 * TIME_STEP) * CLIMB_RATE + ALT_MIN;
elseif mod(time, PERIOD) < 5 * TIME_STEP
    y = (mod(time, PERIOD) - 4 * TIME_STEP) * -CLIMB_RATE + ALT_MIN + STEP_SIZE;
else
    y = ALT_MIN;   % Default option to silence SIMULINK
end

== matlab function X8/Mission Planner/Course Command  ==
  settings: updateMethod=DISCRETE
  data: time input; y output
function y = fcn(time)
%#codegen

TIME_STEP = 30; 
COURSE_INCREMENT = 90; 

y = mod(floor(time/TIME_STEP) * 90, 360) ;

== matlab function X8/Mission Planner/Airspeed Command  ==
  settings: updateMethod=DISCRETE
  data: time input; y output; P parameter
function y = fcn(time,P)
%#codegen
% if time > 100 && time <300 || time>400
% %     y = 12 + 6/50*(time-400);
% y = P.Va + 1+ 2*(sin(1/40*(time-100)*2*pi));
% elseif time >=300 && time<=400
% y = P.Va + 2+ 2*(sin(1/40*(time-100)*2*pi));
% 
% else
    
    y = P.Va;
    if time >300
        y = 22;
    end
    if time<50
        y = 23;
    end
    if time<100 && time>=50
        y = 18;
    end
        
end

== matlab function X8/X1/Forces/MATLAB Function ==
  settings: updateMethod=DISCRETE
  data: states input; tau output; AirData output Bus: AirData; wind input; control input; P parameter; prop_torque output; fault input; stabilityParams input; AerodynamicForces output; controlParams input; prop_rpm output; I_a output; U_out output; time input; faultParams output
function [tau,AirData,prop_torque, AerodynamicForces,prop_rpm,I_a,U_out, faultParams]  = fcn(states,wind,control,P,fault, stabilityParams, controlParams, time)
%#codegen
% ,Va, alpha, beta, course, crab, gamma, gamma_a, wind_b,T_prop
temp = forces([states.Position.p_N,states.Position.p_E,states.Position.p_D, ...
                states.Attitude.phi,states.Attitude.theta,states.Attitude.psi]',...
              [states.Velocity.u,states.Velocity.v,states.Velocity.w, ...
               states.AngularVelocity.p,states.AngularVelocity.q,states.AngularVelocity.r]',...
              [states.Quaternion.ScalarPart;states.Quaternion.VectorPart]',...
              control,  ...
              wind, ...
              P, ...
              fault, ...
              stabilityParams,  ... 
              controlParams, time);
tau = temp(1:6);  % Fx, Fy, Fz, l, m, n in body fixed system
AirData.Va                              = temp(7);
AirData.alpha                           = temp(8);
AirData.beta                            = temp(9);
AirData.Course_angle                    = temp(10);
AirData.Crab_angle                      = temp(11);
AirData.Path_angle                      = temp(12);
AirData.Air_mass_referenced_path_angle  = temp(13);
AirData.wind_x                          = temp(14);
AirData.wind_y                          = temp(15);
AirData.wind_z                          = temp(16);
prop_torque     = temp(17);
AerodynamicForces = temp(18:20);
prop_rpm = temp(21);
I_a = temp(22);
U_out = temp(23);
faultParams = temp(24:end);
%C_L_alpha_n = temp(18:20);

== matlab function X8/X1/Dynamics1/q2euler ==
  data: q input; phi output; theta output; psi output
function [phi,theta,psi] = fcn(q)
%#codegen
[phi,theta,psi] = q2euler(q);
end

== matlab function X8/X1/Dynamics1/dynamics ==
  settings: updateMethod=CONTINUOUS
  data: states input Bus: States; tau input; y output; P parameter
function y = fcn(states,tau, P)
%#codegen

% y = dynamics([states.Position.p_N,states.Position.p_E,states.Position.p_D]', ...
%                 [states.Quaternion.ScalarPart,states.Quaternion.VectorPart']', ...
%                 [states.Velocity.u,states.Velocity.v,states.Velocity.w]',  ...
%                 [states.AngularVelocity.p,states.AngularVelocity.q,states.AngularVelocity.r]', ...
%                 tau, ...
%                 P);
%             
    pos =   [states.Position.p_N,states.Position.p_E,states.Position.p_D]';
    quat = [states.Quaternion.ScalarPart,states.Quaternion.VectorPart']';
    vel = [states.Velocity.u,states.Velocity.v,states.Velocity.w]';
    Omega = [states.AngularVelocity.p,states.AngularVelocity.q,states.AngularVelocity.r]';
            
    gamma = 0; %convergence rate for quaternion normalization
    M_rb = [eye(3) * P.mass,        -P.mass * Smtrx(P.r_cg) ;
            P.mass * Smtrx(P.r_cg),  P.I_cg                 ]; % Fossen 3.44
    %     end
    C_rb = [zeros(3),                                                 -P.mass * Smtrx(vel) - P.mass * Smtrx(Omega) * Smtrx(P.r_cg);
            -P.mass * Smtrx(vel) + P.mass * Smtrx(P.r_cg) * Smtrx(Omega), -Smtrx(P.I_cg * Omega)]; %Fossen 3.56
    
    
    ny_dot = M_rb \ (tau - C_rb * [vel; Omega]);       %(3.20)-(3.21) p 49 in Fossen(2011)
    [~,J1,T] = quatern(quat);
    
    pos_dot = J1 * vel;                                    %(2.69) p30 in Fossen(2011)
    q_dot   = T * Omega - 1/2 * (1 - quat' * quat) * quat;          %(2.73) p31 in Fossen(2011)
    
    y = [pos_dot',q_dot',ny_dot']';
end

== matlab function X8/X1/Calculate Stability Parameters/MATLAB Function1 ==
  settings: updateMethod=CONTINUOUS
  data: states input; alpha output; wind input; beta output
function [alpha,beta] = fcn(states,wind)
v_b = [states.Velocity.u,states.Velocity.v,states.Velocity.w]';
v_r = v_b - wind(1:3);
alpha = atan2(v_r(3),v_r(1));
beta = asin(v_r(2)/sqrt(v_r(1)^2 + v_r(2)^2 + v_r(3)^2));

end

== matlab function X8/Ardupilot SITL send/MATLAB Function2 ==
  data: time_s input; acceleration_lin input; velocity_ang input; velocity_lin input; orientation input; position input; airspeed input
function fcn(time_s, acceleration_lin, velocity_ang, velocity_lin, orientation, position, airspeed)
coder.extrinsic('-sync:on','simSend');
simSend(time_s, velocity_ang, velocity_lin, acceleration_lin, orientation, position, airspeed);
